simulink model "Six_DoF_PID"  (R2020b)
settings: Solver=VariableStepAuto  StartTime=0.0  StopTime=4  RelTol=1e-3
values from neighbouring files (symbols this model uses):
  D = zeros(3,2)    [ss_3DoF_LQR.m]    (also in ss_6DoF_LQR.m = zeros(6,2))
  inertiaxx = 0.0015    [Data_for_simulation.m]
  inertiayy = 0.048    [Data_for_simulation.m]
  inertiazz = 0.048    [Data_for_simulation.m]
  mass = 0.8426    [Data_for_simulation.m]
  moment_arm = 0.29    [Data_for_simulation.m]
undefined symbols (not defined in the file or in its folder): sigbuilder_block
libraries: simulink_extras x3, pid_lib x2, shared6dof x1, aerolibutil x1, vrlib x1, sharedutil x1
settings Model: Creator=raghavendrans  LastModifiedBy=tushark

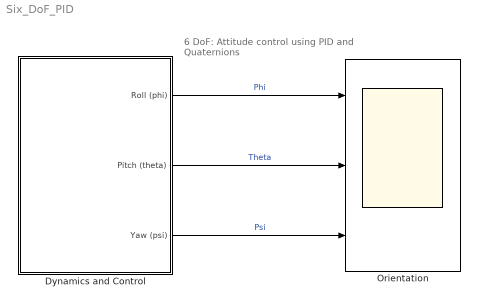
== system Six_DoF_PID ==
  note: 6 DoF: Attitude control using PID and Quaternions
  Dynamics and Control : Subsystem
  Orientation : Scope  NumInputPorts=3
  wires:
  Dynamics and Control/1(Roll (phi)) -> Orientation/1  "Phi"
  Dynamics and Control/2(Pitch (theta)) -> Orientation/2  "Theta"
  Dynamics and Control/3(Yaw (psi)) -> Orientation/3  "Psi"

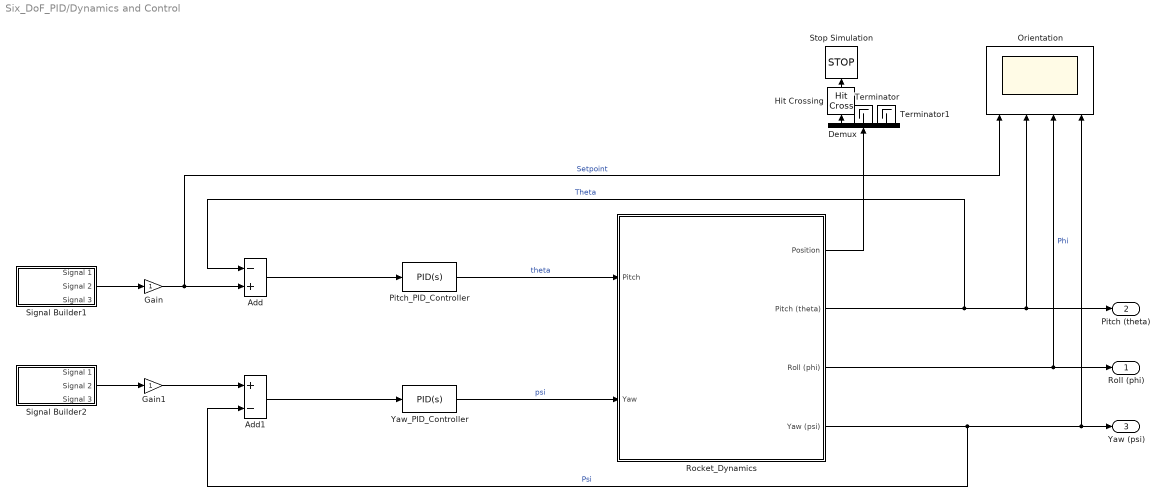
== system Six_DoF_PID/Dynamics and Control ==
  Add : Sum  Inputs=-+
  Add1 : Sum  Inputs=+-
  Demux : Demux  Outputs=3
  Gain : Gain
  Gain1 : Gain
  Hit Crossing : HitCross  HitCrossingDirection=falling
  Orientation : Scope  NumInputPorts=4
  Pitch_PID_Controller : pid_lib/PID Controller  Controller=PID  Form=Parallel  TimeDomain=Continuous-time  UseExternalTs=off  SampleTime=-1  IntegratorMethod=Forward Euler  FilterMethod=Forward Euler  ControllerParametersSource=internal  P=10.75  I=0  D=2.75  UseFilter=on  N=100  TunerSelectOption=Transfer Function Based (PID Tuner App)  InitialConditionSource=internal  InitialConditionForIntegrator=0  InitialConditionForFilter=0  DifferentiatorICPrevScaledInput=0  ExternalReset=none  TrackingMode=off  Kt=1  LimitOutput=on  SatLimitsSource=internal  UpperSaturationLimit=5  LowerSaturationLimit=-5  LinearizeAsGain=on  AntiWindupMode=none  Kb=1  POutMin=[]  POutMax=[]  IOutMin=[]  IOutMax=[]  DOutMin=[]  DOutMax=[]  NOutMin=[]  NOutMax=[]  SumOutMin=[]  SumOutMax=[]  SaturationOutMin=[]  SaturationOutMax=[]  PParamMin=[]  PParamMax=[]  IParamMin=[]  IParamMax=[]  DParamMin=[]  DParamMax=[]  NParamMin=[]  NParamMax=[]  KbParamMin=[]  KbParamMax=[]  KtParamMin=[]  KtParamMax=[]  KbOutMin=[]  KbOutMax=[]  KtOutMin=[]  KtOutMax=[]  IntegratorOutMin=[]  IntegratorOutMax=[]  FilterOutMin=[]  FilterOutMax=[]  SumI1OutMin=[]  SumI1OutMax=[]  SumI2OutMin=[]  SumI2OutMax=[]  SumI3OutMin=[]  SumI3OutMax=[]  SumI4OutMin=[]  SumI4OutMax=[]  SumDOutMin=[]  SumDOutMax=[]  DifferentiatorOutMin=[]  DifferentiatorOutMax=[]  FilterDiffOutCoefMin=[]  FilterDiffOutCoefMax=[]  ReciprocalOutMin=[]  ReciprocalOutMax=[]  SumDenOutMin=[]  SumDenOutMax=[]  SumNumOutMin=[]  SumNumOutMax=[]  DivideOutMin=[]  DivideOutMax=[]  UdiffTsProdOutMin=[]  UdiffTsProdOutMax=[]  NTsProdOutMin=[]  NTsProdOutMax=[]  UintegralTsProdOutMin=[]  UintegralTsProdOutMax=[]  UngainTsProdOutMin=[]  UngainTsProdOutMax=[]  IntegratorContinuousStateAttributes=''  IntegratorStateMustResolveToSignalObject=off  IntegratorRTWStateStorageClass=Auto  FilterContinuousStateAttributes=''  FilterStateMustResolveToSignalObject=off  FilterRTWStateStorageClass=Auto  ParallelPVariant=InternalParameters  IdealPVariant=Disabled  IVariant=InternalParameters  DVariant=InternalParameters  IntegratorVariant=Continuous  SatVariant=Enabled  AWVariant=Passthrough  PCopyVariant=Disabled  TRVariant=Disabled  FdbkBlocksVariant=Forward  IdealPFdbkVariant=Disabled  SatFdbkVariant=Disabled  DerivativeFilterVariant=ContFilter  NVariant=InternalParameters  NCopyVariant=Disabled  FilterICVariant=InternalICsFilter  IntegratorICVariant=InternalICs  ExternalResetVariant=Disabled  TRSumVariant=Passthrough  SumFdbkVariant=Disabled  SumVariant=Sum_PID  TsampFilterVariant=InternalTs  TsampNgainVariant=Passthrough  TsampIntegralVariant=Passthrough  ExternalSaturationOutDataTypeStr=Inherit: Same as second input
  Rocket_Dynamics : Subsystem
  Signal Builder1 : Subsystem  Tag=STV Subsys  LoadFcn=sigbuilder_block('load');  StartFcn=sigbuilder_block('start');  StopFcn=sigbuilder_block('stop');  ClipboardFcn=sigbuilder_block('clipboard');  mask(Sigbuilder block){tuvar=[0:10]}
      mask help: Simulink:masks:SigbuilderBlock_MD
      mask init:
      | if ~strcmp(get_param(bdroot(gcbh),'SimulationStatus'),'stopped') tuvar = sigbuilder_block('maskInit'); end
      settings: CopyFcn=sigbuilder_block('copy');  DeleteFcn=sigbuilder_block('delete');  ModelCloseFcn=sigbuilder_block('modelClose');  PreSaveFcn=sigbuilder_block('preSave');  PauseFcn=sigbuilder_block('pause');  ContinueFcn=sigbuilder_block('continue');  NameChangeFcn=sigbuilder_block('namechange');  OpenFcn=sigbuilder_block('open',[437.6 199.2 550.4 400 ]);  CloseFcn=sigbuilder_block('close');
      mask Display: plot(0, 0, 100, 100,[2, 2, 32, 32, 2], [68, 8, 8, 68, 68],[32, 2], [38, 38], [32, 19, 2],[53, 60, 44], [32, 17, 17, 2],[16, 16, 31, 31]);txt = getActiveGroup(gcbh);text(2, 100, txt,'verticalAlignment', 'top');
  Signal Builder2 : Subsystem  Tag=STV Subsys  LoadFcn=sigbuilder_block('load');  StartFcn=sigbuilder_block('start');  StopFcn=sigbuilder_block('stop');  ClipboardFcn=sigbuilder_block('clipboard');  mask(Sigbuilder block){tuvar=[0:10]}
      mask help: Simulink:masks:SigbuilderBlock_MD
      mask init:
      | if ~strcmp(get_param(bdroot(gcbh),'SimulationStatus'),'stopped') tuvar = sigbuilder_block('maskInit'); end
      settings: CopyFcn=sigbuilder_block('copy');  DeleteFcn=sigbuilder_block('delete');  ModelCloseFcn=sigbuilder_block('modelClose');  PreSaveFcn=sigbuilder_block('preSave');  PauseFcn=sigbuilder_block('pause');  ContinueFcn=sigbuilder_block('continue');  NameChangeFcn=sigbuilder_block('namechange');  OpenFcn=sigbuilder_block('open',[437.6 199.2 550.4 400 ]);  CloseFcn=sigbuilder_block('close');
      mask Display: plot(0, 0, 100, 100,[2, 2, 32, 32, 2], [68, 8, 8, 68, 68],[32, 2], [38, 38], [32, 19, 2],[53, 60, 44], [32, 17, 17, 2],[16, 16, 31, 31]);txt = getActiveGroup(gcbh);text(2, 100, txt,'verticalAlignment', 'top');
  Stop Simulation : Stop
  Terminator : Terminator
  Terminator1 : Terminator
  Yaw_PID_Controller : pid_lib/PID Controller  Controller=PID  Form=Parallel  TimeDomain=Continuous-time  UseExternalTs=off  SampleTime=-1  IntegratorMethod=Forward Euler  FilterMethod=Forward Euler  ControllerParametersSource=internal  P=12.25  I=0  D=3.07  UseFilter=on  N=100  TunerSelectOption=Transfer Function Based (PID Tuner App)  InitialConditionSource=internal  InitialConditionForIntegrator=0  InitialConditionForFilter=0  DifferentiatorICPrevScaledInput=0  ExternalReset=none  TrackingMode=off  Kt=1  LimitOutput=on  SatLimitsSource=internal  UpperSaturationLimit=5  LowerSaturationLimit=-5  LinearizeAsGain=on  AntiWindupMode=none  Kb=1  POutMin=[]  POutMax=[]  IOutMin=[]  IOutMax=[]  DOutMin=[]  DOutMax=[]  NOutMin=[]  NOutMax=[]  SumOutMin=[]  SumOutMax=[]  SaturationOutMin=[]  SaturationOutMax=[]  PParamMin=[]  PParamMax=[]  IParamMin=[]  IParamMax=[]  DParamMin=[]  DParamMax=[]  NParamMin=[]  NParamMax=[]  KbParamMin=[]  KbParamMax=[]  KtParamMin=[]  KtParamMax=[]  KbOutMin=[]  KbOutMax=[]  KtOutMin=[]  KtOutMax=[]  IntegratorOutMin=[]  IntegratorOutMax=[]  FilterOutMin=[]  FilterOutMax=[]  SumI1OutMin=[]  SumI1OutMax=[]  SumI2OutMin=[]  SumI2OutMax=[]  SumI3OutMin=[]  SumI3OutMax=[]  SumI4OutMin=[]  SumI4OutMax=[]  SumDOutMin=[]  SumDOutMax=[]  DifferentiatorOutMin=[]  DifferentiatorOutMax=[]  FilterDiffOutCoefMin=[]  FilterDiffOutCoefMax=[]  ReciprocalOutMin=[]  ReciprocalOutMax=[]  SumDenOutMin=[]  SumDenOutMax=[]  SumNumOutMin=[]  SumNumOutMax=[]  DivideOutMin=[]  DivideOutMax=[]  UdiffTsProdOutMin=[]  UdiffTsProdOutMax=[]  NTsProdOutMin=[]  NTsProdOutMax=[]  UintegralTsProdOutMin=[]  UintegralTsProdOutMax=[]  UngainTsProdOutMin=[]  UngainTsProdOutMax=[]  IntegratorContinuousStateAttributes=''  IntegratorStateMustResolveToSignalObject=off  IntegratorRTWStateStorageClass=Auto  FilterContinuousStateAttributes=''  FilterStateMustResolveToSignalObject=off  FilterRTWStateStorageClass=Auto  ParallelPVariant=InternalParameters  IdealPVariant=Disabled  IVariant=InternalParameters  DVariant=InternalParameters  IntegratorVariant=Continuous  SatVariant=Enabled  AWVariant=Passthrough  PCopyVariant=Disabled  TRVariant=Disabled  FdbkBlocksVariant=Forward  IdealPFdbkVariant=Disabled  SatFdbkVariant=Disabled  DerivativeFilterVariant=ContFilter  NVariant=InternalParameters  NCopyVariant=Disabled  FilterICVariant=InternalICsFilter  IntegratorICVariant=InternalICs  ExternalResetVariant=Disabled  TRSumVariant=Passthrough  SumFdbkVariant=Disabled  SumVariant=Sum_PID  TsampFilterVariant=InternalTs  TsampNgainVariant=Passthrough  TsampIntegralVariant=Passthrough  ExternalSaturationOutDataTypeStr=Inherit: Same as second input
  Roll (phi) : Outport
  Pitch (theta) : Outport  Port=2
  Yaw (psi) : Outport  Port=3
  wires:
  Pitch_PID_Controller/1 -> Rocket_Dynamics/1(Pitch)  "theta"
  Yaw_PID_Controller/1 -> Rocket_Dynamics/2(Yaw)  "psi"
  Add1/1 -> Yaw_PID_Controller/1
  Add/1 -> Pitch_PID_Controller/1
  Rocket_Dynamics/1(Position) -> Demux/1
  Gain1/1 -> Add1/1
  Gain/1 -> Add/2, Orientation/1  "Setpoint"
  Rocket_Dynamics/3(Roll (phi)) -> Roll (phi)/1, Orientation/3  "Phi"
  Rocket_Dynamics/2(Pitch (theta)) -> Pitch (theta)/1, Orientation/2, Add/1  "Theta"
  Rocket_Dynamics/4(Yaw (psi)) -> Yaw (psi)/1, Orientation/4, Add1/2  "Psi"
  Hit Crossing/1 -> Stop Simulation/1
  Demux/3 -> Terminator1/1
  Demux/1 -> Hit Crossing/1
  Demux/2 -> Terminator/1
  Signal Builder1/2(Signal 2) -> Gain/1
  Signal Builder2/2(Signal 2) -> Gain1/1

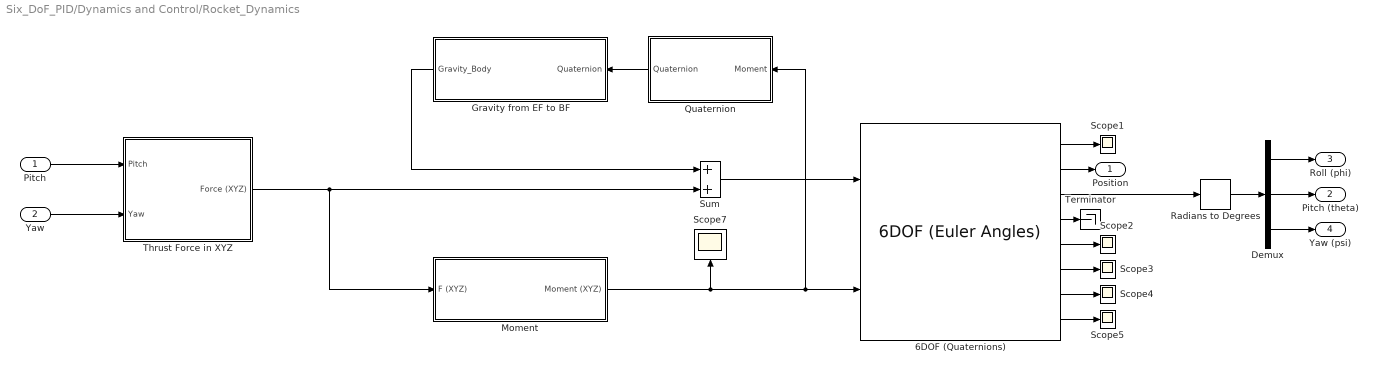
== system Six_DoF_PID/Dynamics and Control/Rocket_Dynamics ==
  Pitch : Inport
  Yaw : Inport  Port=2
  "6DOF (Quaternions) " : shared6dof/6DOF (Euler Angles)  units=Metric (MKS)  mtype=Fixed  rep=Quaternion  xme_0="[150  0 0]"  Vm_0=[0 0 0]  eul_0=[0 0 0]  pm_0=[0 0 0]  mass_0=mass  mass_e=0.5  mass_f=2.0  inertia=[inertiaxx inertiayy inertiazz].*eye(3)  inertia_e=eye(3)  inertia_f=2*eye(3)  k_quat=1.0  vre_flag=on  abi_flag=off  aMode=0  xme_statename=''  Vm_statename=''  eul_statename=''  quat_statename=''  pm_statename=''  mass_statename=''
      settings: SourceProductBaseCode=AE,PW,MT,UV,VE,VP
  Demux : Demux  Outputs=3
  "Gravity from EF to BF " : Subsystem
  Moment : Subsystem
  Quaternion : Subsystem
  Radians to Degrees : simulink_extras/Transformations/Radians to Degrees
  Scope{1..5,7} (6 alike) : Scope
  Sum : Sum
  Terminator : Terminator
  Thrust Force in XYZ : Subsystem
  Position : Outport
  Pitch (theta) : Outport  Port=2
  Roll (phi) : Outport  Port=3
  Yaw (psi) : Outport  Port=4
  wires:
  "6DOF (Quaternions) "/1 -> Scope1/1
  Pitch/1 -> Thrust Force in XYZ/1(Pitch)
  Demux/3 -> Yaw (psi)/1
  Demux/2 -> Pitch (theta)/1
  "6DOF (Quaternions) "/7 -> Scope4/1
  Moment/1(Moment (XYZ)) -> Quaternion/1(Moment), "6DOF (Quaternions) "/2, Scope7/1
  Sum/1 -> "6DOF (Quaternions) "/1
  "6DOF (Quaternions) "/5 -> Scope2/1
  "6DOF (Quaternions) "/8 -> Scope5/1
  "6DOF (Quaternions) "/2 -> Position/1
  Thrust Force in XYZ/1(Force (XYZ)) -> Moment/1(F (XYZ)), Sum/2
  Yaw/1 -> Thrust Force in XYZ/2(Yaw)
  Demux/1 -> Roll (phi)/1
  Radians to Degrees/1 -> Demux/1
  "Gravity from EF to BF "/1(Gravity_Body) -> Sum/1
  "6DOF (Quaternions) "/6 -> Scope3/1
  "6DOF (Quaternions) "/3 -> Radians to Degrees/1
  "6DOF (Quaternions) "/4 -> Terminator/1
  Quaternion/1(Quaternion) -> "Gravity from EF to BF "/1(Quaternion)

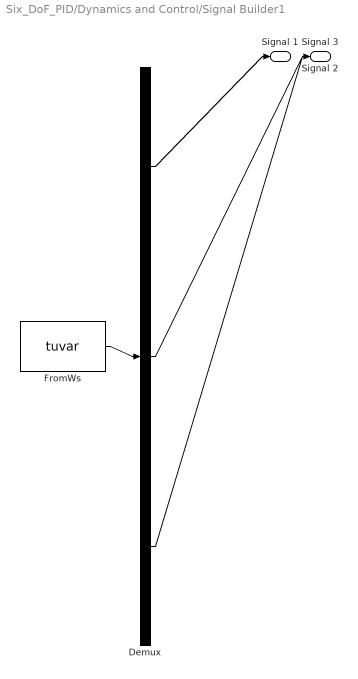
== system Six_DoF_PID/Dynamics and Control/Signal Builder1 ==
  Demux : Demux  Tag=STV Demux  Outputs=3
      settings: DisplayOption=none
  FromWs : FromWorkspace  Tag=STV FromWs  VariableName=tuvar
      SigBuilderData=|
      | common.afterFinalStr = 'Extrapolate'
      | common.sampleTime = 0
      | dataSet.timeRange = [0 10]
      | dataSet.name = 'Group 1'
      | sbobj.Groups.Name = 'Group 1'
      | sbobj.Groups.Signals(1).Name = 'Signal 1'
      | sbobj.Groups.Signals(1).XData = [0 10]
      | sbobj.Groups.Signals(1).YData = [5 5]
      | sbobj.Groups.Signals(2).Name = 'Signal 2'
      | sbobj.Groups.Signals(2).XData = [0 1 1 10]
      | sbobj.Groups.Signals(2).YData = [5 5 0 0]
      | sbobj.Groups.Signals(3).Name = 'Signal 3'
      | sbobj.Groups.Signals(3).XData = [0 1 1 10]
      | sbobj.Groups.Signals(3).YData = [0 0 5 5]
  Signal 1 : Outport  Tag=STV Outport
  Signal 2 : Outport  Tag=STV Outport  Port=2
  Signal 3 : Outport  Tag=STV Outport  Port=3
  wires:
  Demux/1 -> Signal 1/1
  Demux/2 -> Signal 2/1
  Demux/3 -> Signal 3/1
  FromWs/1 -> Demux/1

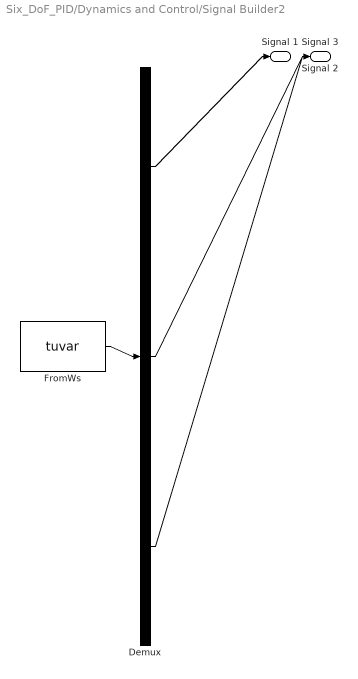
== system Six_DoF_PID/Dynamics and Control/Signal Builder2 ==
  Demux : Demux  Tag=STV Demux  Outputs=3
      settings: DisplayOption=none
  FromWs : FromWorkspace  Tag=STV FromWs  VariableName=tuvar
      SigBuilderData=|
      | common.afterFinalStr = 'Extrapolate'
      | common.sampleTime = 0
      | dataSet.timeRange = [0 10]
      | dataSet.name = 'Group 1'
      | sbobj.Groups.Name = 'Group 1'
      | sbobj.Groups.Signals(1).Name = 'Signal 1'
      | sbobj.Groups.Signals(1).XData = [0 10]
      | sbobj.Groups.Signals(1).YData = [5 5]
      | sbobj.Groups.Signals(2).Name = 'Signal 2'
      | sbobj.Groups.Signals(2).XData = [0 1 1 10]
      | sbobj.Groups.Signals(2).YData = [5 5 0 0]
      | sbobj.Groups.Signals(3).Name = 'Signal 3'
      | sbobj.Groups.Signals(3).XData = [0 1 1 10]
      | sbobj.Groups.Signals(3).YData = [0 0 5 5]
  Signal 1 : Outport  Tag=STV Outport
  Signal 2 : Outport  Tag=STV Outport  Port=2
  Signal 3 : Outport  Tag=STV Outport  Port=3
  wires:
  Demux/1 -> Signal 1/1
  Demux/2 -> Signal 2/1
  Demux/3 -> Signal 3/1
  FromWs/1 -> Demux/1

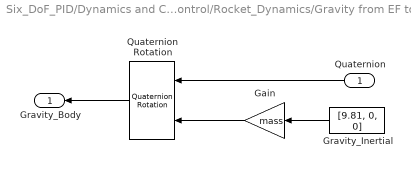
== system Six_DoF_PID/Dynamics and Control/Rocket_Dynamics/Gravity from EF to BF  ==
  Quaternion : Inport
  Gain : Gain  Gain=mass
  Gravity_Inertial : Constant  Value=[9.81, 0, 0]
  Quaternion Rotation : aerolibutil/Quaternion Rotation
  Gravity_Body : Outport
  wires:
  Gravity_Inertial/1 -> Gain/1
  Gain/1 -> Quaternion Rotation/2
  Quaternion Rotation/1 -> Gravity_Body/1
  Quaternion/1 -> Quaternion Rotation/1

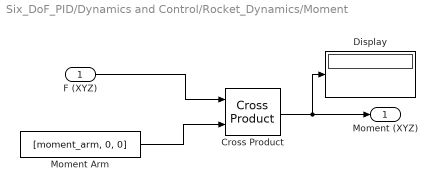
== system Six_DoF_PID/Dynamics and Control/Rocket_Dynamics/Moment ==
  F (XYZ) : Inport
  Cross Product : vrlib/Utilities/Cross Product
  Display : Display
  Moment Arm : Constant  Value=[moment_arm, 0, 0]
  Moment (XYZ) : Outport
  wires:
  Cross Product/1 -> Display/1, Moment (XYZ)/1
  Moment Arm/1 -> Cross Product/2
  F (XYZ)/1 -> Cross Product/1

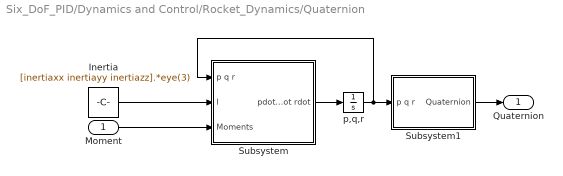
== system Six_DoF_PID/Dynamics and Control/Rocket_Dynamics/Quaternion ==
  Moment : Inport  Unit=N*m  PortDimensions=3
  Inertia : Constant  Value=[inertiaxx inertiayy inertiazz].*eye(3)
  Subsystem : Subsystem
  Subsystem1 : Subsystem
  p,q,r : Integrator
  Quaternion : Outport  VectorParamsAs1DForOutWhenUnconnected=off
  wires:
  p,q,r/1 -> Subsystem1/1(p q r), Subsystem/1(p q r)
  Subsystem1/1(Quaternion) -> Quaternion/1
  Moment/1 -> Subsystem/3(Moments)
  Inertia/1 -> Subsystem/2(I)
  Subsystem/1(pdot qdot rdot) -> p,q,r/1

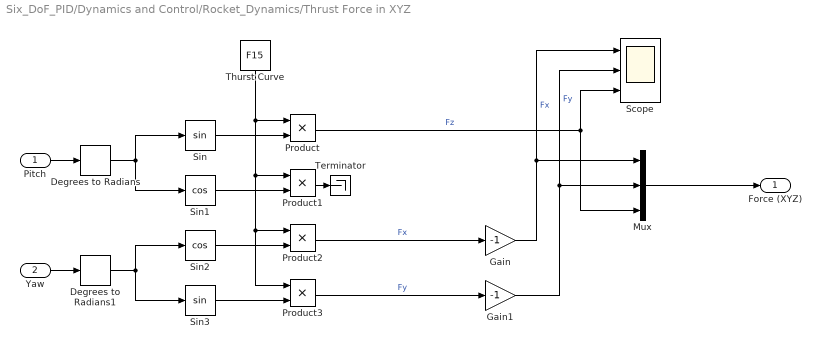
== system Six_DoF_PID/Dynamics and Control/Rocket_Dynamics/Thrust Force in XYZ ==
  Pitch : Inport
  Yaw : Inport  Port=2
  Degrees to Radians : simulink_extras/Transformations/Degrees to Radians
  Degrees to Radians1 : simulink_extras/Transformations/Degrees to Radians
  Gain : Gain  Gain=-1
  Gain1 : Gain  Gain=-1
  Mux : Mux  Inputs=3
  Product{,1..3} (4 alike) : Product
  Scope : Scope  NumInputPorts=3
  Sin : Trigonometry
  Sin1 : Trigonometry  Operator=cos
  Sin2 : Trigonometry  Operator=cos
  Sin3 : Trigonometry
  Terminator : Terminator
  Thurst Curve : FromWorkspace  VariableName=F15
  Force (XYZ) : Outport
  wires:
  Sin2/1 -> Product2/2
  Sin/1 -> Product/2
  Sin1/1 -> Product1/2
  Product3/1 -> Gain1/1  "Fy"
  Product/1 -> Mux/3, Scope/3  "Fz"
  Thurst Curve/1 -> Product/1, Product1/1, Product2/1, Product3/1
  Mux/1 -> Force (XYZ)/1
  Sin3/1 -> Product3/2
  Pitch/1 -> Degrees to Radians/1
  Yaw/1 -> Degrees to Radians1/1
  Gain/1 -> Scope/1, Mux/1  "Fx"
  Degrees to Radians1/1 -> Sin3/1, Sin2/1
  Degrees to Radians/1 -> Sin/1, Sin1/1
  Gain1/1 -> Mux/2, Scope/2  "Fy"
  Product2/1 -> Gain/1  "Fx"
  Product1/1 -> Terminator/1

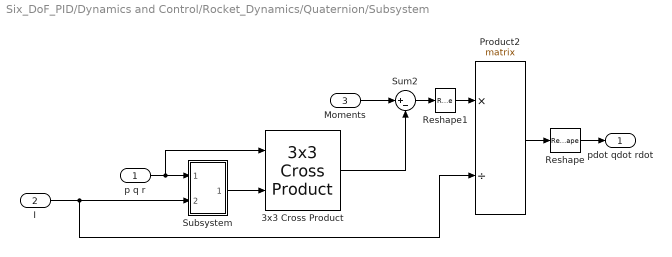
== system Six_DoF_PID/Dynamics and Control/Rocket_Dynamics/Quaternion/Subsystem ==
  p q r : Inport
  I : Inport  Port=2
  Moments : Inport  Port=3
  3x3 Cross Product : sharedutil/3x3 Cross Product  aMode=aMode
      settings: SourceProductBaseCode=AE,PW,MT,UV,VE,VP
  Product2 : Product  Inputs=*/  Multiplication=Matrix(*)  SaturateOnIntegerOverflow=on  OutDataTypeStr=Inherit: Same as first input
  Reshape : Reshape
  Reshape1 : Reshape  OutputDimensionality=Row vector (2-D)
  Subsystem : Subsystem
  Sum2 : Sum  Inputs=|+-  SaturateOnIntegerOverflow=on
  pdot qdot rdot : Outport  VectorParamsAs1DForOutWhenUnconnected=off
  wires:
  Moments/1 -> Sum2/1
  Reshape1/1 -> Product2/1
  I/1 -> Subsystem/2(Inertia), Product2/2
  Sum2/1 -> Reshape1/1
  p q r/1 -> Subsystem/1(p q r), 3x3 Cross Product/1
  Product2/1 -> Reshape/1
  Reshape/1 -> pdot qdot rdot/1
  Subsystem/1(I * w) -> 3x3 Cross Product/2
  3x3 Cross Product/1 -> Sum2/2

== system Six_DoF_PID/Dynamics and Control/Rocket_Dynamics/Quaternion/Subsystem1 ==
  p q r : Inport
  Subsystem : Subsystem
  q0 q1 q2 q3 : Integrator  InitialCondition=[1, 0, 0, 0]
  Quaternion : Outport  VectorParamsAs1DForOutWhenUnconnected=off
  wires:
  Subsystem/1(qdot) -> q0 q1 q2 q3/1
  p q r/1 -> Subsystem/1(p q r1)
  q0 q1 q2 q3/1 -> Subsystem/2(q0 q1 q2 q3), Quaternion/1

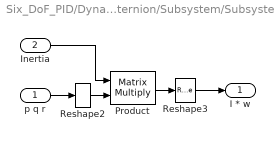
== system Six_DoF_PID/Dynamics and Control/Rocket_Dynamics/Quaternion/Subsystem/Subsystem ==
  p q r : Inport
  Inertia : Inport  Port=2
  Product : Product  Multiplication=Matrix(*)  InputSameDT=on  SaturateOnIntegerOverflow=on  OutDataTypeStr=Inherit: Same as first input
  Reshape2 : Reshape  OutputDimensionality=Column vector (2-D)
  Reshape3 : Reshape
  I * w : Outport  VectorParamsAs1DForOutWhenUnconnected=off
  wires:
  p q r/1 -> Reshape2/1
  Product/1 -> Reshape3/1
  Inertia/1 -> Product/1
  Reshape2/1 -> Product/2
  Reshape3/1 -> I * w/1

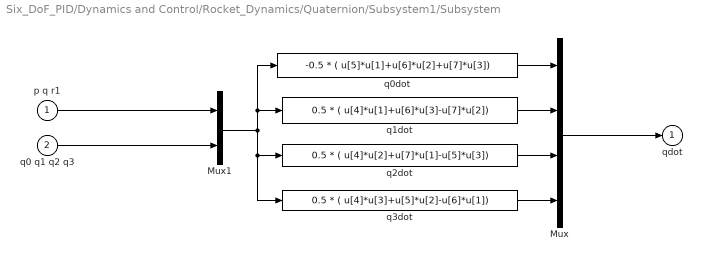
== system Six_DoF_PID/Dynamics and Control/Rocket_Dynamics/Quaternion/Subsystem1/Subsystem ==
  p q r1 : Inport
  q0 q1 q2 q3 : Inport  Port=2  PortDimensions=4
  Mux : Mux
  Mux1 : Mux  Inputs=[3 4]
  q0dot : Fcn  Expr=-0.5 * ( u[5]*u[1]+u[6]*u[2]+u[7]*u[3])
  q1dot : Fcn  Expr=0.5 * ( u[4]*u[1]+u[6]*u[3]-u[7]*u[2])
  q2dot : Fcn  Expr=0.5 * ( u[4]*u[2]+u[7]*u[1]-u[5]*u[3])
  q3dot : Fcn  Expr=0.5 * ( u[4]*u[3]+u[5]*u[2]-u[6]*u[1])
  qdot : Outport  InitialOutput=0  VectorParamsAs1DForOutWhenUnconnected=off
  wires:
  Mux/1 -> qdot/1
  Mux1/1 -> q0dot/1, q1dot/1, q3dot/1, q2dot/1
  p q r1/1 -> Mux1/1
  q0 q1 q2 q3/1 -> Mux1/2
  q0dot/1 -> Mux/1
  q1dot/1 -> Mux/2
  q2dot/1 -> Mux/3
  q3dot/1 -> Mux/4
